simulink model "Final_V620140905h5b_fuben1"  (Simulink 7.9)
settings: Solver=FixedStepDiscrete  StartTime=0.0  StopTime=1  FixedStep=Auto  RelTol=1e-3
undefined symbols (not defined in the file or in its folder): Down, Up
libraries: tiiqmathlib x157, idelinklib_common x83, c2833xlib x37, simulink x12, c28xdmclib x12, c280xlib x7, simulink_extras x4, commutil2 x2, idelinklib_tgtpref x1, idelinklib_ticcs x1
(part 2 of 7)

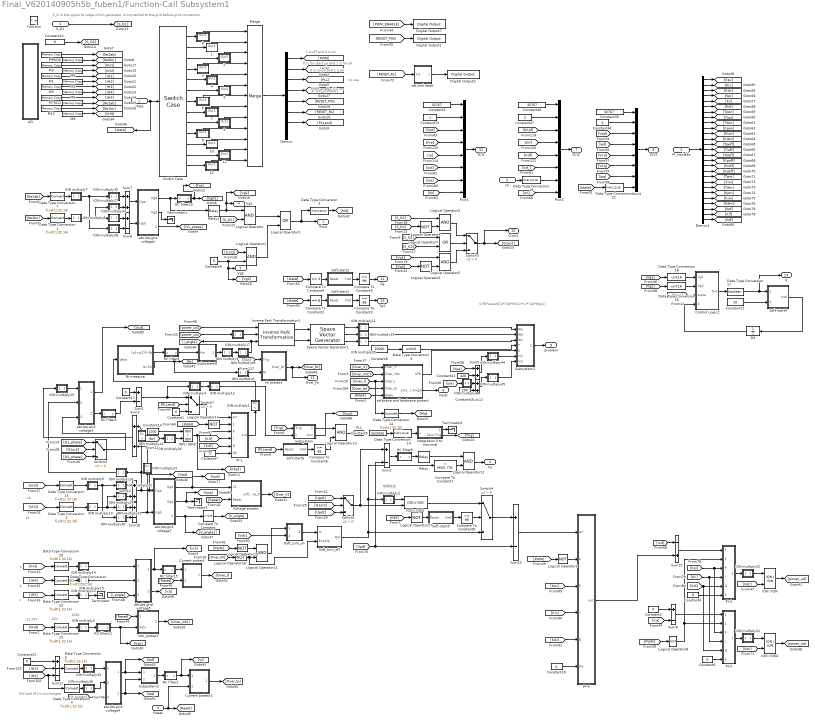
== system Final_V620140905h5b_fuben1/Function-Call Subsystem1 ==
  note: 1 is off and 0 is on
  note: 0 is for start up and 1 is for pll
  note: 0 is no pll and 1 is pll
  note: 21.25V
  note: 42V
  note: 1656
  note: PWM enable 1 is on
  note: S_G is the signal to judge which generator is connected to the grid before grid connection
  note: a
  note: b
  note: c
  note: no use
  note: IH2 and IH1 is exchanged.
  note: 0.95*squart[(2*740*Md)2+(2*740*Mq)2]
  note: cb
  note: ac
  note: 电网软启
  state : Inport
  PI_variable : Inport  Port=2
  Reset : Inport  Port=3
  S_G1 : Inport  Port=4
  ch : Inport  Port=5
  function : TriggerPort  TriggerType=function-call
  0 : Subsystem  TreatAsAtomicUnit=on
  1 : Subsystem  TreatAsAtomicUnit=on
  10 : Subsystem  TreatAsAtomicUnit=on
  11 : Subsystem  TreatAsAtomicUnit=on
  12 : Subsystem  TreatAsAtomicUnit=on
  2 : Subsystem  TreatAsAtomicUnit=on
  3 : Subsystem  TreatAsAtomicUnit=on
  4 : Subsystem  TreatAsAtomicUnit=on
  5 : Subsystem  TreatAsAtomicUnit=on
  6 : Subsystem  TreatAsAtomicUnit=on
  7 : Subsystem  TreatAsAtomicUnit=on
  8 : Subsystem  TreatAsAtomicUnit=on
  9 : Subsystem  TreatAsAtomicUnit=on
  AD : Subsystem  Priority=1
  Compare To Constant : simulink/Logic and Bit Operations/Compare To Constant  relop=>  const=0.8  OutDataTypeStr=uint8
  Compare To Constant1 : simulink/Logic and Bit Operations/Compare To Constant  relop=>  const=560/1.732  OutDataTypeStr=uint8
  Compare To Constant2 : simulink/Logic and Bit Operations/Compare To Constant  relop===  const=8  OutDataTypeStr=boolean
  Compare To Constant3 : simulink/Logic and Bit Operations/Compare To Constant  relop=>=  const=99  OutDataTypeStr=boolean
  Compare To Constant4 : simulink/Logic and Bit Operations/Compare To Constant  relop===  const=3  OutDataTypeStr=boolean
  Compare To Constant5 : simulink/Logic and Bit Operations/Compare To Constant  relop=>=  const=99  OutDataTypeStr=boolean
  Compare To Constant6 : simulink/Logic and Bit Operations/Compare To Constant  relop=>=  const=99  OutDataTypeStr=boolean
  Compare To Constant9 : simulink/Logic and Bit Operations/Compare To Constant  relop=<=  const=99  OutDataTypeStr=boolean
  Constant{1..2,4,6..7,17..18} (7 alike) : Constant  Value=0  OutDataTypeStr=fixdt(1,32,16)
  Constant11 : Constant  Value=10  OutDataTypeStr=fixdt(1,32,16)
  Constant12 : Constant  Value=0  OutDataTypeStr=boolean
  Constant13 : Constant  OutDataTypeStr=fixdt(1,32,16)
  Constant14 : Constant  Value=1200  OutDataTypeStr=fixdt(1,32,16)
  Constant16 : Constant  Value=100  OutDataTypeStr=fixdt(1,32,16)
  Constant21 : Constant  Value=420  OutDataTypeStr=fixdt(1,32,16)
  Constant23 : Constant  Value=0  OutDataTypeStr=fixdt(1,32,16)  SampleTime=-1
  Constant3 : Constant  Value=32767  OutDataTypeStr=fixdt(1,32,16)
  Constant30 : Constant  Value=32767  OutDataTypeStr=fixdt(1,32,16)
  Constant44 : Constant  Value=3  OutDataTypeStr=fixdt(1,32,16)
  Constant46 : Constant  Value=32767  OutDataTypeStr=fixdt(1,32,16)
  Constant47 : Constant  Value=2  OutDataTypeStr=fixdt(1,32,16)
  Constant5 : Constant  Value=50/5000  OutDataTypeStr=double
  Constant8 : Constant  Value=15000  OutDataTypeStr=int16
  Constant9 : Constant  Value=0  OutDataTypeStr=Inherit: Inherit via back propagation
  Control Logic2 : Stateflow chart  TreatAsAtomicUnit=on
  Current protect : Subsystem
  Current protect1 : Subsystem
  D5 : UnitDelay  SampleTime=-1
  Data Type Conversion{1..2,4..7,12..15,19..23} (15 alike) : DataTypeConversion  OutDataTypeStr=fixdt(1,32,16)
  Data Type Conversion16 : DataTypeConversion  OutDataTypeStr=uint16
  Data Type Conversion17 : DataTypeConversion  OutDataTypeStr=boolean
  Data Type Conversion18 : DataTypeConversion  OutDataTypeStr=uint16
  Data Type Conversion3 : DataTypeConversion  OutDataTypeStr=uint16
  Demux : Demux  Outputs=8
  Demux1 : Demux  Outputs=27
  Digital Output1 : c2833xlib/Digital Output  Priority=1  GPIO_Number=GPIO48~GPIO55  GPIO_Bit0=off  GPIO_BIT0_Toggle=off  GPIO_Bit1=on  GPIO_BIT1_Toggle=off  GPIO_Bit2=off  GPIO_BIT2_Toggle=off  GPIO_Bit3=off  GPIO_BIT3_Toggle=off  GPIO_Bit4=off  GPIO_BIT4_Toggle=off  GPIO_Bit5=off  GPIO_BIT5_Toggle=off  GPIO_Bit6=off  GPIO_BIT6_Toggle=off  GPIO_Bit7=off  GPIO_BIT7_Toggle=off
  Digital Output2 : c2833xlib/Digital Output  Priority=1  GPIO_Number=GPIO48~GPIO55  GPIO_Bit0=on  GPIO_BIT0_Toggle=off  GPIO_Bit1=off  GPIO_BIT1_Toggle=off  GPIO_Bit2=off  GPIO_BIT2_Toggle=off  GPIO_Bit3=off  GPIO_BIT3_Toggle=off  GPIO_Bit4=off  GPIO_BIT4_Toggle=off  GPIO_Bit5=off  GPIO_BIT5_Toggle=off  GPIO_Bit6=off  GPIO_BIT6_Toggle=off  GPIO_Bit7=off  GPIO_BIT7_Toggle=off
  Digital Output7 : c2833xlib/Digital Output  Priority=1  GPIO_Number=GPIO16~GPIO23  GPIO_Bit0=off  GPIO_BIT0_Toggle=off  GPIO_Bit1=off  GPIO_BIT1_Toggle=off  GPIO_Bit2=off  GPIO_BIT2_Toggle=off  GPIO_Bit3=on  GPIO_BIT3_Toggle=off  GPIO_Bit4=off  GPIO_BIT4_Toggle=off  GPIO_Bit5=off  GPIO_BIT5_Toggle=off  GPIO_Bit6=off  GPIO_BIT6_Toggle=off  GPIO_Bit7=off  GPIO_BIT7_Toggle=off
  ION multiply1 : Subsystem  mask{x=1/50}
      mask prompts: x "gain"
  ION multiply10 : Subsystem  mask{x=0.02536*50/29.6/1.0181}
      mask prompts: x "gain"
  ION multiply11 : Subsystem  mask{x=-1}
      mask prompts: x "gain"
  ION multiply12 : Subsystem  mask{x=1/100}
      mask prompts: x "gain"
  ION multiply13 : Subsystem  mask{x=0.0086*75/38}
      mask prompts: x "gain"
  ION multiply14 : Subsystem  mask{x=0.0086*75/38}
      mask prompts: x "gain"
  ION multiply15 : Subsystem  mask{x=0.0086*75/38}
      mask prompts: x "gain"
  ION multiply16 : Subsystem  mask{x=-1}
      mask prompts: x "gain"
  ION multiply17 : Subsystem  mask{x=-1}
      mask prompts: x "gain"
  ION multiply19 : Subsystem  mask{x=-1}
      mask prompts: x "gain"
  ION multiply2 : Subsystem  mask{x=1/327}
      mask prompts: x "gain"
  ION multiply20 : Subsystem  mask{x=-1}
      mask prompts: x "gain"
  ION multiply21 : Subsystem  mask{x=750/1000}
      mask prompts: x "gain"
  ION multiply22 : Subsystem  mask{x=750/1000}
      mask prompts: x "gain"
  ION multiply23 : Subsystem  mask{x=-1}
      mask prompts: x "gain"
  ION multiply24 : Subsystem  mask{x=-1}
      mask prompts: x "gain"
  ION multiply25 : Subsystem  mask{x=-1}
      mask prompts: x "gain"
  ION multiply26 : Subsystem  mask{x=10}
      mask prompts: x "gain"
  ION multiply27 : Subsystem  mask{x=1/3}
      mask prompts: x "gain"
  ION multiply28 : Subsystem  mask{x=1/3}
      mask prompts: x "gain"
  ION multiply29 : Subsystem  mask{x=1/3}
      mask prompts: x "gain"
  ION multiply3 : Subsystem  mask{x=0.04016*305/298}
      mask prompts: x "gain"
  ION multiply30 : Subsystem  mask{x=1/3}
      mask prompts: x "gain"
  ION multiply31 : Subsystem  mask{x=1/3}
      mask prompts: x "gain"
  ION multiply32 : Subsystem  mask{x=2/3}
      mask prompts: x "gain"
  ION multiply33 : Subsystem  mask{x=-0.0086*75/38}
      mask prompts: x "gain"
  ION multiply34 : Subsystem  mask{x=1/3}
      mask prompts: x "gain"
  ION multiply35 : Subsystem  mask{x=2/3}
      mask prompts: x "gain"
  ION multiply36 : Subsystem  mask{x=-0.0086*75/38}
      mask prompts: x "gain"
  ION multiply39 : Subsystem  mask{x=1/100}
      mask prompts: x "gain"
  ION multiply4 : Subsystem  mask{x=1/50}
      mask prompts: x "gain"
  ION multiply44 : Subsystem  mask{x=1/8}
      mask prompts: x "gain"
  ION multiply45 : Subsystem  mask{x=0}
      mask prompts: x "gain"
  ION multiply46 : Subsystem  mask{x=-1}
      mask prompts: x "gain"
  ION multiply5 : Subsystem  mask{x=1/50}
      mask prompts: x "gain"
  ION multiply6 : Subsystem  mask{x=10}
      mask prompts: x "gain"
  ION multiply7 : Subsystem  mask{x=-0.02436}
      mask prompts: x "gain"
  ION multiply8 : Subsystem  mask{x=-0.02436}
      mask prompts: x "gain"
  ION multiply9 : Subsystem  mask{x=0.02536*50/29.6/1.0181}
      mask prompts: x "gain"
  IQN / IQN : tiiqmathlib/IQN // IQN
  IQN / IQN2 : tiiqmathlib/IQN // IQN
  IQN / IQN3 : tiiqmathlib/IQN // IQN
  IQN x IQN1 : tiiqmathlib/IQN x IQN  multiplyOption=Multiply
  Integration 0 to maximal : Subsystem  mask{a=1}
      mask prompts: a "the maximal y"
  Inverse Park Transformation1 : c28xdmclib/Inverse Park Transformation
  Logical Operator{,1,3,5,11..13} (7 alike) : Logic  AllPortsSameDT=off  OutDataTypeStr=boolean
  Logical Operator{8..10,14,16} (5 alike) : Logic  Operator=NOT  Inputs=1  AllPortsSameDT=off  OutDataTypeStr=boolean
  Logical Operator17 : Logic  Operator=NOT  AllPortsSameDT=off  OutDataTypeStr=boolean
  Logical Operator2 : Logic  Operator=OR  AllPortsSameDT=off  OutDataTypeStr=boolean
  Logical Operator4 : Logic  Operator=NOT  AllPortsSameDT=off  OutDataTypeStr=boolean
  Logical Operator6 : Logic  Operator=NOT  AllPortsSameDT=off  OutDataTypeStr=boolean
  Logical Operator7 : Logic  Operator=OR  AllPortsSameDT=off  OutDataTypeStr=boolean
  M1 : idelinklib_common/Memory Copy  Priority=2  copyFrom=Specified source code symbol  copyFromAddressSource=Specify via dialog  copyFromAddress=M1  copyFromSrcCode=M1  dataTypeFrom=int16  dataDimensionFrom=1  useOffsetFrom=off  offsetFromSrc=Specify via dialog  offsetFrom=0  strideFrom=1  copyTo=Output port  copyToAddressSource=Specify via dialog  copyToAddress=temp  copyToSrcCode=M7  dataTypeTo=int16  useOffsetTo=on  offsetToSrc=Specify via dialog  offsetTo=0  strideTo=1  sampleTime=inf  useInitValue=off  initValueSrc=Specify constant value  initValue=bin2dec('00000000')  initValueSrcCode=myInitValueVariable  useAsMask=off  maskOperator=bitwise AND  useTermValue=off  termValue=bin2dec('00000000')  isRealtimeEnabled=off  emitCCBeforeWrite=off  CCBeforeWrite=/* Custom Code Before Write*/  emitCCAfterWrite=off  CCAfterWrite=/* Custom Code After Write*/  useDMACopy=off  enableBlockingMode=off
  M10 : idelinklib_common/Memory Copy  Priority=2  copyFrom=Specified source code symbol  copyFromAddressSource=Specify via dialog  copyFromAddress=M1  copyFromSrcCode=M10  dataTypeFrom=int16  dataDimensionFrom=1  useOffsetFrom=off  offsetFromSrc=Specify via dialog  offsetFrom=0  strideFrom=1  copyTo=Output port  copyToAddressSource=Specify via dialog  copyToAddress=temp  copyToSrcCode=M7  dataTypeTo=int16  useOffsetTo=on  offsetToSrc=Specify via dialog  offsetTo=0  strideTo=1  sampleTime=inf  useInitValue=off  initValueSrc=Specify constant value  initValue=bin2dec('00000000')  initValueSrcCode=myInitValueVariable  useAsMask=off  maskOperator=bitwise AND  useTermValue=off  termValue=bin2dec('00000000')  isRealtimeEnabled=off  emitCCBeforeWrite=off  CCBeforeWrite=/* Custom Code Before Write*/  emitCCAfterWrite=off  CCAfterWrite=/* Custom Code After Write*/  useDMACopy=off  enableBlockingMode=off
  M11 : idelinklib_common/Memory Copy  Priority=2  copyFrom=Specified source code symbol  copyFromAddressSource=Specify via dialog  copyFromAddress=M1  copyFromSrcCode=M11  dataTypeFrom=int16  dataDimensionFrom=1  useOffsetFrom=off  offsetFromSrc=Specify via dialog  offsetFrom=0  strideFrom=1  copyTo=Output port  copyToAddressSource=Specify via dialog  copyToAddress=temp  copyToSrcCode=M7  dataTypeTo=int16  useOffsetTo=on  offsetToSrc=Specify via dialog  offsetTo=0  strideTo=1  sampleTime=inf  useInitValue=off  initValueSrc=Specify constant value  initValue=bin2dec('00000000')  initValueSrcCode=myInitValueVariable  useAsMask=off  maskOperator=bitwise AND  useTermValue=off  termValue=bin2dec('00000000')  isRealtimeEnabled=off  emitCCBeforeWrite=off  CCBeforeWrite=/* Custom Code Before Write*/  emitCCAfterWrite=off  CCAfterWrite=/* Custom Code After Write*/  useDMACopy=off  enableBlockingMode=off
  M12 : idelinklib_common/Memory Copy  Priority=2  copyFrom=Specified source code symbol  copyFromAddressSource=Specify via dialog  copyFromAddress=M1  copyFromSrcCode=M12  dataTypeFrom=int16  dataDimensionFrom=1  useOffsetFrom=off  offsetFromSrc=Specify via dialog  offsetFrom=0  strideFrom=1  copyTo=Output port  copyToAddressSource=Specify via dialog  copyToAddress=temp  copyToSrcCode=M7  dataTypeTo=int16  useOffsetTo=on  offsetToSrc=Specify via dialog  offsetTo=0  strideTo=1  sampleTime=inf  useInitValue=off  initValueSrc=Specify constant value  initValue=bin2dec('00000000')  initValueSrcCode=myInitValueVariable  useAsMask=off  maskOperator=bitwise AND  useTermValue=off  termValue=bin2dec('00000000')  isRealtimeEnabled=off  emitCCBeforeWrite=off  CCBeforeWrite=/* Custom Code Before Write*/  emitCCAfterWrite=off  CCAfterWrite=/* Custom Code After Write*/  useDMACopy=off  enableBlockingMode=off
  M2 : idelinklib_common/Memory Copy  Priority=2  copyFrom=Specified source code symbol  copyFromAddressSource=Specify via dialog  copyFromAddress=M1  copyFromSrcCode=M2  dataTypeFrom=int16  dataDimensionFrom=1  useOffsetFrom=off  offsetFromSrc=Specify via dialog  offsetFrom=0  strideFrom=1  copyTo=Output port  copyToAddressSource=Specify via dialog  copyToAddress=temp  copyToSrcCode=M7  dataTypeTo=int16  useOffsetTo=on  offsetToSrc=Specify via dialog  offsetTo=0  strideTo=1  sampleTime=inf  useInitValue=off  initValueSrc=Specify constant value  initValue=bin2dec('00000000')  initValueSrcCode=myInitValueVariable  useAsMask=off  maskOperator=bitwise AND  useTermValue=off  termValue=bin2dec('00000000')  isRealtimeEnabled=off  emitCCBeforeWrite=off  CCBeforeWrite=/* Custom Code Before Write*/  emitCCAfterWrite=off  CCAfterWrite=/* Custom Code After Write*/  useDMACopy=off  enableBlockingMode=off
  M3 : idelinklib_common/Memory Copy  Priority=2  copyFrom=Specified source code symbol  copyFromAddressSource=Specify via dialog  copyFromAddress=M1  copyFromSrcCode=M3  dataTypeFrom=int16  dataDimensionFrom=1  useOffsetFrom=off  offsetFromSrc=Specify via dialog  offsetFrom=0  strideFrom=1  copyTo=Output port  copyToAddressSource=Specify via dialog  copyToAddress=temp  copyToSrcCode=M7  dataTypeTo=int16  useOffsetTo=on  offsetToSrc=Specify via dialog  offsetTo=0  strideTo=1  sampleTime=inf  useInitValue=off  initValueSrc=Specify constant value  initValue=bin2dec('00000000')  initValueSrcCode=myInitValueVariable  useAsMask=off  maskOperator=bitwise AND  useTermValue=off  termValue=bin2dec('00000000')  isRealtimeEnabled=off  emitCCBeforeWrite=off  CCBeforeWrite=/* Custom Code Before Write*/  emitCCAfterWrite=off  CCAfterWrite=/* Custom Code After Write*/  useDMACopy=off  enableBlockingMode=off
  M4 : idelinklib_common/Memory Copy  Priority=2  copyFrom=Specified source code symbol  copyFromAddressSource=Specify via dialog  copyFromAddress=M1  copyFromSrcCode=M4  dataTypeFrom=int16  dataDimensionFrom=1  useOffsetFrom=off  offsetFromSrc=Specify via dialog  offsetFrom=0  strideFrom=1  copyTo=Output port  copyToAddressSource=Specify via dialog  copyToAddress=temp  copyToSrcCode=M7  dataTypeTo=int16  useOffsetTo=on  offsetToSrc=Specify via dialog  offsetTo=0  strideTo=1  sampleTime=inf  useInitValue=off  initValueSrc=Specify constant value  initValue=bin2dec('00000000')  initValueSrcCode=myInitValueVariable  useAsMask=off  maskOperator=bitwise AND  useTermValue=off  termValue=bin2dec('00000000')  isRealtimeEnabled=off  emitCCBeforeWrite=off  CCBeforeWrite=/* Custom Code Before Write*/  emitCCAfterWrite=off  CCAfterWrite=/* Custom Code After Write*/  useDMACopy=off  enableBlockingMode=off
  M5 : idelinklib_common/Memory Copy  Priority=2  copyFrom=Specified source code symbol  copyFromAddressSource=Specify via dialog  copyFromAddress=M1  copyFromSrcCode=M5  dataTypeFrom=int16  dataDimensionFrom=1  useOffsetFrom=off  offsetFromSrc=Specify via dialog  offsetFrom=0  strideFrom=1  copyTo=Output port  copyToAddressSource=Specify via dialog  copyToAddress=temp  copyToSrcCode=M7  dataTypeTo=int16  useOffsetTo=on  offsetToSrc=Specify via dialog  offsetTo=0  strideTo=1  sampleTime=inf  useInitValue=off  initValueSrc=Specify constant value  initValue=bin2dec('00000000')  initValueSrcCode=myInitValueVariable  useAsMask=off  maskOperator=bitwise AND  useTermValue=off  termValue=bin2dec('00000000')  isRealtimeEnabled=off  emitCCBeforeWrite=off  CCBeforeWrite=/* Custom Code Before Write*/  emitCCAfterWrite=off  CCAfterWrite=/* Custom Code After Write*/  useDMACopy=off  enableBlockingMode=off
  M6 : idelinklib_common/Memory Copy  Priority=2  copyFrom=Specified source code symbol  copyFromAddressSource=Specify via dialog  copyFromAddress=M1  copyFromSrcCode=M6  dataTypeFrom=int16  dataDimensionFrom=1  useOffsetFrom=off  offsetFromSrc=Specify via dialog  offsetFrom=0  strideFrom=1  copyTo=Output port  copyToAddressSource=Specify via dialog  copyToAddress=temp  copyToSrcCode=M7  dataTypeTo=int16  useOffsetTo=on  offsetToSrc=Specify via dialog  offsetTo=0  strideTo=1  sampleTime=inf  useInitValue=off  initValueSrc=Specify constant value  initValue=bin2dec('00000000')  initValueSrcCode=myInitValueVariable  useAsMask=off  maskOperator=bitwise AND  useTermValue=off  termValue=bin2dec('00000000')  isRealtimeEnabled=off  emitCCBeforeWrite=off  CCBeforeWrite=/* Custom Code Before Write*/  emitCCAfterWrite=off  CCAfterWrite=/* Custom Code After Write*/  useDMACopy=off  enableBlockingMode=off
  M7 : idelinklib_common/Memory Copy  Priority=2  copyFrom=Specified source code symbol  copyFromAddressSource=Specify via dialog  copyFromAddress=M1  copyFromSrcCode=M7  dataTypeFrom=int16  dataDimensionFrom=1  useOffsetFrom=off  offsetFromSrc=Specify via dialog  offsetFrom=0  strideFrom=1  copyTo=Output port  copyToAddressSource=Specify via dialog  copyToAddress=temp  copyToSrcCode=M7  dataTypeTo=int16  useOffsetTo=on  offsetToSrc=Specify via dialog  offsetTo=0  strideTo=1  sampleTime=inf  useInitValue=off  initValueSrc=Specify constant value  initValue=bin2dec('00000000')  initValueSrcCode=myInitValueVariable  useAsMask=off  maskOperator=bitwise AND  useTermValue=off  termValue=bin2dec('00000000')  isRealtimeEnabled=off  emitCCBeforeWrite=off  CCBeforeWrite=/* Custom Code Before Write*/  emitCCAfterWrite=off  CCAfterWrite=/* Custom Code After Write*/  useDMACopy=off  enableBlockingMode=off
  M8 : idelinklib_common/Memory Copy  Priority=2  copyFrom=Specified source code symbol  copyFromAddressSource=Specify via dialog  copyFromAddress=M1  copyFromSrcCode=M8  dataTypeFrom=int16  dataDimensionFrom=1  useOffsetFrom=off  offsetFromSrc=Specify via dialog  offsetFrom=0  strideFrom=1  copyTo=Output port  copyToAddressSource=Specify via dialog  copyToAddress=temp  copyToSrcCode=M7  dataTypeTo=int16  useOffsetTo=on  offsetToSrc=Specify via dialog  offsetTo=0  strideTo=1  sampleTime=inf  useInitValue=off  initValueSrc=Specify constant value  initValue=bin2dec('00000000')  initValueSrcCode=myInitValueVariable  useAsMask=off  maskOperator=bitwise AND  useTermValue=off  termValue=bin2dec('00000000')  isRealtimeEnabled=off  emitCCBeforeWrite=off  CCBeforeWrite=/* Custom Code Before Write*/  emitCCAfterWrite=off  CCAfterWrite=/* Custom Code After Write*/  useDMACopy=off  enableBlockingMode=off
  M9 : idelinklib_common/Memory Copy  Priority=2  copyFrom=Specified source code symbol  copyFromAddressSource=Specify via dialog  copyFromAddress=M1  copyFromSrcCode=M9  dataTypeFrom=int16  dataDimensionFrom=1  useOffsetFrom=off  offsetFromSrc=Specify via dialog  offsetFrom=0  strideFrom=1  copyTo=Output port  copyToAddressSource=Specify via dialog  copyToAddress=temp  copyToSrcCode=M7  dataTypeTo=int16  useOffsetTo=on  offsetToSrc=Specify via dialog  offsetTo=0  strideTo=1  sampleTime=inf  useInitValue=off  initValueSrc=Specify constant value  initValue=bin2dec('00000000')  initValueSrcCode=myInitValueVariable  useAsMask=off  maskOperator=bitwise AND  useTermValue=off  termValue=bin2dec('00000000')  isRealtimeEnabled=off  emitCCBeforeWrite=off  CCBeforeWrite=/* Custom Code Before Write*/  emitCCAfterWrite=off  CCAfterWrite=/* Custom Code After Write*/  useDMACopy=off  enableBlockingMode=off
  Merge : Merge  Inputs=13
  Mux1 : Mux  Inputs=8
  Mux2 : Mux  Inputs=8
  Mux3 : Mux  Inputs=8
  Nr measure : Subsystem
  Nr protect : Subsystem
  PI-1 : Subsystem  mask{ermax=200, ermin=-200, max=150, min=-150}
      mask prompts: ermax "Err max limit"; ermin "Err min limit"; max "Output max limit"; min "Output min limit"
  PI-3 : Subsystem  mask{ermax=500, ermin=-500, max=500, min=-500}
      mask prompts: ermax "Err max limit"; ermin "Err min limit"; max "Output max limit"; min "Output min limit"
  PI-4 : Subsystem  mask{ermax=500, ermin=-500, max=165, min=0}
      mask prompts: ermax "Err max limit"; ermin "Err min limit"; max "Output max limit"; min "Output min limit"
  PI-5 : Subsystem  mask{ermax=500, ermin=-500, max=500, min=-500}
      mask prompts: ermax "Err max limit"; ermin "Err min limit"; max "Output max limit"; min "Output min limit"
  RC filter10 : Subsystem  mask{a=0.01}
      mask prompts: a "Time Constant"
  RC filter11 : Subsystem  mask{a=0.01}
      mask prompts: a "Time Constant"
  RC filter15 : Subsystem  mask{a=0.1}
      mask prompts: a "Time Constant"
  RC filter2 : Subsystem  mask{a=0.5}
      mask prompts: a "Time Constant"
  RC filter3 : Subsystem  mask{a=0.5}
      mask prompts: a "Time Constant"
  RC filter4 : Subsystem  mask{a=0.8}
      mask prompts: a "Time Constant"
  RC filter9 : Subsystem  mask{a=0.8}
      mask prompts: a "Time Constant"
  Relay : Relay  OnSwitchValue=20  OffSwitchValue=10  OnOutputValue=0  OffOutputValue=1
  Relay1 : Relay  OnSwitchValue=300  OffSwitchValue=250
  Soft-start1 : Subsystem  mask{a=0.02/0.2, b=100}
      mask prompts: a "soft time"; b "Vref"
  Soft-start2 : Subsystem  mask{a=0.02/0.01, b=100}
      mask prompts: a "soft time"; b "Vref"
  Soft-start4 : Subsystem
  Soft-start5 : Subsystem  mask{a=0.02/2, b=100}
      mask prompts: a "soft time"; b "Vref"
  Soft-start6 : Subsystem  mask{a=0.02/6, b=100}
      mask prompts: a "soft time"; b "Vref"
  Soft_turn_off : Subsystem
  Soft_turn_on : Subsystem
  Space Vector Generator1 : c28xdmclib/Space Vector Generator
  Subsystem : Subsystem
  Subsystem1 : Subsystem
  Subsystem2 : Subsystem
  Subsystem8 : Subsystem
  Sum{1..2,6,9..10,13} (6 alike) : Sum  Inputs=+-
  Sum{3,5,7,12,17} (5 alike) : Sum
  Sum15 : Sum  Inputs=-+
  Sum21 : Sum  Inputs=+--
  Switch Case : SwitchCase  CaseConditions={0,1,2,3,4,5,6,7,8,9,10,11,12}  ShowDefaultCase=off
  Switch{1..4,7} (5 alike) : Switch  Criteria=u2 > Threshold  SaturateOnIntegerOverflow=on  InputSameDT=on
  Terminator{,1..3} (4 alike) : Terminator
  Vdc_protect : Subsystem
  Voltage protect : Subsystem
  abc/dq-grid voltage1 : Subsystem
  abc/dq-grid voltage3 : Subsystem
  abc/dq-grid voltage4 : Subsystem
  abc/dq-grid voltage5 : Subsystem
  abc/dq-grid voltage7 : Subsystem
  set and reset : Subsystem
  softwave and hardwave protect : Subsystem
  Vbus : Outport
  Vs : Outport  Port=2
  PLL : Outport  Port=3
  Vg1 : Outport  Port=4
  Vg2 : Outport  Port=5
  Fault : Outport  Port=6
  SCI2 : Outport  Port=7
  SCI3 : Outport  Port=8
  problem : Outport  Port=9
  G1or2 : Outport  Port=10
  Sg : Outport  Port=11
  SCI1 : Outport  Port=12
  Over_Nr : Outport  Port=13
  K : Outport  Port=14
  Sg1 : Outport  Port=15
  wires:
  Inverse Park Transformation1/1 -> Space Vector Generator1/1
  Inverse Park Transformation1/2 -> Space Vector Generator1/2
  Subsystem8/1(angle) -> ION multiply5/1(x)
  [No1ab] -> Data Type Conversion7/1
  [No1bc] -> Data Type Conversion1/1
  abc/dq-grid voltage1/1(Ugd) -> RC filter10/1(x), Relay1/1
  Switch Case/1 -> 0/Action
  1/1(Out1) -> Merge/2
  2/1(Out1) -> Merge/3
  3/1(Out1) -> Merge/4
  4/1(Out1) -> Merge/5
  5/1(Out1) -> Merge/6
  Merge/1 -> Demux/1
  Demux/1 -> [PWM]
  Demux/2 -> [REF]
  state/1 -> Switch Case/1, [state]
  Demux/3 -> [PLL]
  Relay1/1 -> Logical Operator/1, Vg1/1, [Vg1]
  [S_G1] -> Logical Operator/2
  Logical Operator/1 -> Logical Operator2/1
  Logical Operator2/1 -> Vbus/1, Data Type Conversion5/1
  Constant12/1 -> [S_G2]
  [S_G1] -> Logical Operator3/1
  Logical Operator4/1 -> Logical Operator3/2
  [S_G2] -> Logical Operator4/1
  [G1or2] -> Switch1/2
  [Ugd2] -> Switch1/3
  [Ugd1] -> Switch1/1
  [Vg1] -> Logical Operator5/1
  Logical Operator6/1 -> Logical Operator5/2
  [Vg2] -> Logical Operator6/1
  Switch3/1 -> [G1or2], G1or2/1
  Logical Operator7/1 -> Switch3/2
  [S_G1] -> Logical Operator7/1
  [S_G2] -> Logical Operator7/2
  6/1(Out1) -> Merge/7
  Logical Operator3/1 -> Switch3/1
  Logical Operator5/1 -> Switch3/3
  Data Type Conversion1/1 -> ION multiply8/1(x)
  Data Type Conversion7/1 -> ION multiply7/1(x)
  [PWM_ENABLE] -> Digital Output7/1
  Demux/4 -> [PWM_ENABLE]
  [RESET_PIN] -> Digital Output1/1
  Demux/5 -> [RESET_PIN]
  Demux/6 -> [RESET_RL]
  Space Vector Generator1/1 -> ION multiply11/1(x)
  Space Vector Generator1/2 -> ION multiply19/1(x)
  Space Vector Generator1/3 -> ION multiply20/1(x)
  Data Type Conversion2/1 -> ION multiply10/1(x)
  Data Type Conversion13/1 -> ION multiply9/1(x)
  ION multiply10/1(Kx) -> ION multiply29/1(x), ION multiply31/1(x)
  [VH2] -> Data Type Conversion13/1
  [VH1] -> Data Type Conversion2/1
  [IH3] -> Data Type Conversion20/1
  [IH4] -> Data Type Conversion21/1
  Data Type Conversion21/1 -> ION multiply13/1(x)
  Data Type Conversion20/1 -> ION multiply14/1(x)
  [IH5] -> Data Type Conversion23/1
  Data Type Conversion23/1 -> ION multiply15/1(x)
  abc/dq-grid voltage5/1(igd) -> RC filter15/1(x), [icd]
  [i_angle] -> abc/dq-grid voltage5/3(angle)
  RC filter15/1(y) -> Current protect/1(igdin)
  7/1(Out1) -> Merge/8
  Mux2/1 -> SCI2/1
  Constant30/1 -> Mux3/1
  Constant44/1 -> Mux3/2
  Mux3/1 -> SCI3/1
  Constant46/1 -> Mux2/1
  Constant47/1 -> Mux2/2
  Subsystem1/1(Out1) -> problem/1
  [on] -> Mux2/8
  Switch4/1 -> Sum13/1
  Voltage protect/1(softwave_V) -> [Over_V]
  [Reset] -> Voltage protect/2(Reset)
  [Reset] -> Current protect/2(Reset)
  Current protect/1(Software_I) -> [Over_I]
  Sum2/1 -> RC filter9/1(x)
  RC filter9/1(y) -> Relay/1
  Constant5/1 -> Data Type Conversion14/1
  Data Type Conversion14/1 -> Integration 0 to maximal/1(x)
  Integration 0 to maximal/2(Zero Trig) -> [Trig]
  [Over_V] -> softwave and hardwave protect/1(Over_V)
  RC filter10/1(y) -> [Ugd1], [Fre]
  [VH9] -> Data Type Conversion15/1
  Data Type Conversion15/1 -> ION multiply3/1(x)
  ION multiply3/1(Kx) -> RC filter11/1(x)
  RC filter11/1(y) -> Vdc_protect/2(Vdin), [Vdc]
  [Over_Vdc] -> softwave and hardwave protect/2(Over_Vdc)
  Compare To Constant/1 -> [V_angle]
  [Reset] -> Vdc_protect/1(Reset)
  Vdc_protect/1(Vdguoya) -> [Over_Vdc]
  Switch Case/9 -> 8/Action
  8/1(Out1) -> Merge/9
  Switch Case/8 -> 7/Action
  Switch Case/7 -> 6/Action
  Switch Case/6 -> 5/Action
  Switch Case/5 -> 4/Action
  Switch Case/4 -> 3/Action
  Switch Case/3 -> 2/Action
  Switch Case/2 -> 1/Action
  Demux/7 -> [PLLend]
  Switch Case/10 -> 9/Action
  9/1(Out1) -> Merge/10
  0/1(Out1) -> Merge/1
  10/1(Out1) -> Merge/11
  11/1(Out1) -> Merge/12
  Switch Case/12 -> 11/Action
  Switch Case/13 -> 12/Action
  12/1(Out1) -> Merge/13
  [Over_I] -> softwave and hardwave protect/3(Over_I), Data Type Conversion12/1
  abc/dq-grid voltage5/2(igq) -> [icq]
  ION multiply14/1(Kx) -> abc/dq-grid voltage5/1(iga)
  ION multiply13/1(Kx) -> abc/dq-grid voltage5/2(igb)
  ION multiply15/1(Kx) -> Terminator/1
  M1/1 -> [IH1]
  M2/1 -> [IH2]
  M3/1 -> [VH1]
  M4/1 -> [VH2]
  M5/1 -> [IH3]
  M6/1 -> [IH4]
  M7/1 -> [IH5]
  M8/1 -> [VH9]
  M11/1 -> [No1ab]
  M12/1 -> [No1bc]
  M9/1 -> [No2ab]
  M10/1 -> [No2bc]
  ION multiply11/1(Kx) -> Subsystem1/1(Wa)
  ION multiply19/1(Kx) -> Subsystem1/2(Wb)
  ION multiply20/1(Kx) -> Subsystem1/3(Wc)
  PI-3/1(out) -> ION multiply21/1(x)
  ION multiply21/1(Kx) -> IQN / IQN2/1
  ION multiply32/1(Kx) -> Sum12/1
  ION multiply29/1(Kx) -> Sum12/2
  ION multiply31/1(Kx) -> Sum10/1
  ION multiply30/1(Kx) -> Sum10/2
  Sum12/1 -> ION multiply16/1(x), ION multiply24/1(x), abc/dq-grid voltage7/1(Uga), [Vpa]
  Sum10/1 -> abc/dq-grid voltage7/2(Ugb), ION multiply23/1(x)
  abc/dq-grid voltage7/3(Phase) -> Compare To Constant/1, [V_angle1]
  abc/dq-grid voltage7/2(Ugq) -> Terminator3/1, [Vpq]
  Integration 0 to maximal/1(y) -> Terminator2/1
  [Vpd] -> Mux3/3
  [ipd] -> Mux3/4
  [Vcq] -> Mux3/6
  [ipq] -> Mux3/7
  abc/dq-grid voltage7/1(Ugd) -> Voltage protect/1(V1), [Vpd]
  [Vcd] -> Mux3/5
  [power_uq] -> ION multiply17/1(x)
  [power_ud] -> Inverse Park Transformation1/1
  [PWM] -> Logical Operator9/1
  Logical Operator10/1 -> Logical Operator11/1
  [PWM] -> Logical Operator10/1
  Switch1/1 -> IQN x IQN1/2, Sum2/1
  ION multiply2/1(Kx) -> IQN x IQN1/1
  IQN x IQN1/1 -> Switch4/1
  ION multiply22/1(Kx) -> IQN / IQN/1
  Logical Operator8/1 -> PI-5/2(reset), PI-3/2(reset)
  [PWM] -> Logical Operator8/1
  [Vdc] -> Soft_turn_on/2(Vdc)
  Switch Case/11 -> 10/Action
  set and reset/1(Out1) -> Digital Output2/1
  [RESET_RL] -> set and reset/1(In1)
  IQN / IQN/1 -> [power_ud]
  IQN / IQN2/1 -> [power_uq]
  [icd] -> Sum15/1
  [icq] -> Sum9/2
  PI-5/1(out) -> ION multiply22/1(x)
  Nr measure/2(Nr/10) -> [Nr], ION multiply6/1(x)
  [Kpi] -> PI-5/3(P), PI-3/3(P)
  [Kii] -> PI-5/4(I), PI-3/4(I)
  [Kdi] -> PI-5/5(D), PI-3/5(D)
  Sum15/1 -> PI-5/1(err)
  Sum9/1 -> PI-3/1(err)
  Compare To Constant1/1 -> Logical Operator12/2
  Logical Operator12/1 -> Vs/1
  Relay/1 -> Logical Operator12/1
  Logical Operator9/1 -> PI-4/2(reset)
  PI_variable/1 -> Demux1/1
  Demux1/1 -> [Kpv]
  Demux1/2 -> [Kiv]
  Demux1/3 -> [Kdv]
  Demux1/4 -> [Kpi]
  Demux1/5 -> [Kii]
  Demux1/6 -> [Kdi]
  Demux1/7 -> [Tpon]
  Demux1/8 -> [Tion]
  Demux1/9 -> [Tdon]
  Demux1/10 -> [Kpon]
  Demux1/11 -> [Kion]
  Demux1/12 -> [Kdon]
  Demux1/13 -> [Tpoff]
  Demux1/14 -> [Tioff]
  Demux1/15 -> [Tdoff]
  Demux1/16 -> [Kpoff]
  Demux1/17 -> [Kioff]
  Demux1/18 -> [Kdoff]
  Demux1/19 -> [Tpm]
  Demux1/20 -> [Tim]
  Demux1/21 -> [Tdm]
  Demux1/22 -> [Kpm]
  Demux1/23 -> [Kim]
  Demux1/24 -> [Kdm]
  Constant4/1 -> PI-5/6(OV)
  Constant6/1 -> PI-3/6(OV)
  Demux1/25 -> [Kpf]
  Demux1/26 -> [Kif]
  Demux1/27 -> [Kdf]
  Constant8/1 -> Data Type Conversion3/1
  [G1or2] -> Switch2/2
  [G1_phase] -> Switch2/1
  [G2_phase] -> Switch2/3
  Data Type Conversion3/1 -> Subsystem1/4(T)
  [Over_Ip] -> softwave and hardwave protect/4(Over_Ip)
  Constant2/1 -> Sum9/1
  Soft-start2/1(Vref) -> Compare To Constant5/1
  [state] -> Compare To Constant4/1
  Compare To Constant4/1 -> Soft-start2/1(Reset)
  Compare To Constant5/1 -> Sg/1
  [Vdc] -> IQN / IQN/2
  [Vdc] -> IQN / IQN2/2
  ION multiply9/1(Kx) -> ION multiply32/1(x), ION multiply30/1(x)
  [Vpd] -> Sum13/2, Sum2/2
  ION multiply8/1(Kx) -> ION multiply34/1(x), ION multiply27/1(x)
  ION multiply35/1(Kx) -> Sum7/1
  ION multiply27/1(Kx) -> Sum7/2
  ION multiply34/1(Kx) -> Sum6/1
  ION multiply28/1(Kx) -> Sum6/2
  Sum7/1 -> abc/dq-grid voltage1/1(Uga)
  Sum6/1 -> abc/dq-grid voltage1/2(Ugb)
  ION multiply7/1(Kx) -> ION multiply28/1(x), ION multiply35/1(x)
  abc/dq-grid voltage1/3(Phase) -> [G1_phase]
  abc/dq-grid voltage1/2(Ugq) -> Terminator1/1
  Sum13/1 -> PI-4/1(err)
  [PWM] -> Logical Operator14/1
  abc/dq-grid voltage4/1(igd) -> Subsystem2/1(In1), [ipd]
  abc/dq-grid voltage4/2(igq) -> Subsystem2/2(In2), [ipq]
  Current protect1/1(Software_I) -> [Over_Ip]
  RC filter2/1(y) -> Current protect1/1(igdin), [ip]
  PI-4/1(out) -> Sum15/2
  Subsystem2/1(Out1) -> RC filter2/1(x)
  Nr measure/1((p1+p2)Fr-Fp) -> RC filter4/1(x)
  [KKpf] -> Mux2/3
  [Kif] -> Mux2/4
  [Kdf] -> Mux2/5
  [icd_] -> Mux2/6
  Mux1/1 -> SCI1/1
  Constant3/1 -> Mux1/1
  Constant13/1 -> Mux1/2
  [Nr] -> Mux1/8
  [Vpd] -> Mux1/3
  [ip] -> Mux1/5
  [ipd] -> Mux1/6
  [ipq] -> Mux1/7
  [V_angle1] -> abc/dq-grid voltage4/3(angle)
  [Fre] -> Mux1/4
  ION multiply6/1(Kx) -> Nr protect/2(Nr)
  Reset/1 -> [Reset], Current protect1/2(Reset)
  Data Type Conversion5/1 -> [Md]
  [Trig] -> Nr protect/1(Trig)
  Nr protect/1(Over_Nr) -> [Over_Nr], Over_Nr/1
  Soft_turn_on/1(Out) -> Soft_turn_off/1(In)
  Soft_turn_off/1(Ref) -> Compare To Constant1/1, ION multiply2/1(x), Switch4/3
  [Over_Nr] -> Logical Operator16/1
  [PWM] -> softwave and hardwave protect/5(PWM)
  softwave and hardwave protect/2(protect singal) -> Fault/1
  Logical Operator11/1 -> Soft_turn_on/1(Enable)
  Logical Operator16/1 -> Logical Operator11/2, Soft_turn_off/2(Enable)
  S_G1/1 -> [S_G1]
  Constant11/1 -> Soft-start4/2(T)
  Control Logic2/1(Out) -> Data Type Conversion17/1
  Soft-start4/1(Vref) -> D5/1
  D5/1 -> Control Logic2/4(K)
  [state] -> Control Logic2/3(state)
  [Vg1] -> Data Type Conversion18/1
  [Vg2] -> Data Type Conversion16/1
  Data Type Conversion18/1 -> Control Logic2/1(Vg1)
  Data Type Conversion16/1 -> Control Logic2/2(Vg2)
  Data Type Conversion17/1 -> Soft-start4/1(Reset), K/1
  Data Type Conversion12/1 -> [Mq]
  ch/1 -> Data Type Conversion19/1
  Soft-start5/1(Vref) -> Compare To Constant9/1
  Logical Operator17/1 -> Soft-start5/1(Reset)
  [REF] -> Logical Operator17/1
  Compare To Constant9/1 -> Switch4/2
  Data Type Conversion19/1 -> Mux2/7
  Soft-start1/1(Vref) -> Compare To Constant3/1
  [state] -> Compare To Constant2/1
  Compare To Constant2/1 -> Soft-start1/1(Reset)
  Compare To Constant3/1 -> Sg1/1
  [state] -> Data Type Conversion22/1
  Data Type Conversion22/1 -> Mux3/8
  RC filter4/1(y) -> Subsystem8/1(fre)
  ION multiply5/1(Kx) -> ION multiply39/1(x)
  ION multiply39/1(Kx) -> Inverse Park Transformation1/3, [i_angle]
  Switch2/1 -> abc/dq-grid voltage3/3(angle)
  Logical Operator14/1 -> PI-1/2(reset)
  Constant17/1 -> Sum1/1
  Sum1/1 -> Switch7/1, ION multiply4/1(x)
  Constant1/1 -> Switch7/3
  abc/dq-grid voltage3/2(igq) -> RC filter3/1(x)
  [PLLend] -> Switch7/2
  Switch7/1 -> PI-1/1(err)
  PI-1/1(out) -> ION multiply1/1(x)
  abc/dq-grid voltage3/1(igd) -> [Vcd]
  Constant7/1 -> PI-1/6(OV)
  Constant9/1 -> Logical Operator1/2, Vg2/1, [Vg2]
  [S_G2] -> Logical Operator1/1
  Logical Operator1/1 -> Logical Operator2/2
  [Trig] -> Subsystem/1(Trig)
  Subsystem/1(On/off) -> Logical Operator13/1
  Logical Operator13/1 -> PLL/1
  Compare To Constant6/1 -> Logical Operator13/2
  Soft-start6/1(Vref) -> Compare To Constant6/1
  [PLLend] -> Soft-start6/1(Reset)
  RC filter3/1(y) -> Sum1/2
  ION multiply1/1(Kx) -> Nr measure/1(deta)
  Subsystem/2(sum) -> [Vcq]
  ION multiply4/1(Kx) -> ION multiply12/1(x)
  ION multiply12/1(Kx) -> Subsystem/2(x)
  ION multiply16/1(Kx) -> abc/dq-grid voltage3/2(igb)
  ION multiply23/1(Kx) -> Sum3/2
  ION multiply24/1(Kx) -> Sum3/1
  Sum3/1 -> ION multiply25/1(x)
  ION multiply25/1(Kx) -> abc/dq-grid voltage3/1(iga)
  [Kif] -> PI-1/4(I)
  [Kdf] -> PI-1/5(D)
  Constant14/1 -> IQN / IQN3/1
  [Nr] -> ION multiply26/1(x)
  ION multiply26/1(Kx) -> IQN / IQN3/2
  IQN / IQN3/1 -> PI-1/3(P), [KKpf]
  Data Type Conversion4/1 -> ION multiply36/1(x)
  Data Type Conversion6/1 -> ION multiply33/1(x)
  Constant23/1 -> Sum21/1
  [IH1] -> Sum21/2
  [IH2] -> Sum21/3, Data Type Conversion4/1
  Sum21/1 -> Data Type Conversion6/1
  ION multiply33/1(Kx) -> abc/dq-grid voltage4/1(iga)
  ION multiply36/1(Kx) -> abc/dq-grid voltage4/2(igb)
  ION multiply17/1(Kx) -> Inverse Park Transformation1/2
  softwave and hardwave protect/1(SFB) -> Subsystem1/5(SFB)
  Sum5/1 -> ION multiply44/1(x)
  Sum17/1 -> ION multiply45/1(x)
  Constant21/1 -> Sum5/2
  [Vpa] -> Sum5/1
  [ipa] -> ION multiply46/1(x)
  ION multiply46/1(Kx) -> Sum17/1
  Constant16/1 -> Sum17/2
  ION multiply44/1(Kx) -> Subsystem1/6(In1)
  ION multiply45/1(Kx) -> Subsystem1/7(In2)
  Constant18/1 -> PI-4/6(OV)
  [Kdv] -> PI-4/5(D)
  [Kiv] -> PI-4/4(I)
  [Kpv] -> PI-4/3(P)

== system Final_V620140905h5b_fuben1/Function-Call Subsystem3 ==
  function : TriggerPort  TriggerType=function-call
  Constant10 : Constant  OutDataTypeStr=fixdt(1,32,16)
  Integration 0 to maximal3 : Subsystem  mask{a=4}
      mask prompts: a "the maximal y"
  Memory Copy1 : idelinklib_common/Memory Copy  Priority=9  copyFrom=Specified source code symbol  copyFromAddressSource=Specify via dialog  copyFromAddress=hex2dec('200004')  copyFromSrcCode=data1  dataTypeFrom=int16  dataDimensionFrom=8  useOffsetFrom=off  offsetFromSrc=Specify via dialog  offsetFrom=0  strideFrom=1  copyTo=Output port  copyToAddressSource=Specify via dialog  copyToAddress=temp  copyToSrcCode=wave3  dataTypeTo=int16  useOffsetTo=off  offsetToSrc=Input port  offsetTo=0  strideTo=1  sampleTime=inf  useInitValue=off  initValueSrc=Specify constant value  initValue=bin2dec('00000000')  initValueSrcCode=myInitValueVariable  useAsMask=off  maskOperator=bitwise AND  useTermValue=off  termValue=bin2dec('00000000')  isRealtimeEnabled=off  emitCCBeforeWrite=off  CCBeforeWrite=/* Custom Code Before Write*/  emitCCAfterWrite=off  CCAfterWrite=/* Custom Code After Write*/  useDMACopy=off  enableBlockingMode=off
  Memory Copy2 : idelinklib_common/Memory Copy  Priority=9  copyFrom=Specified source code symbol  copyFromAddressSource=Specify via dialog  copyFromAddress=hex2dec('200004')  copyFromSrcCode=data2  dataTypeFrom=int16  dataDimensionFrom=8  useOffsetFrom=off  offsetFromSrc=Specify via dialog  offsetFrom=0  strideFrom=1  copyTo=Output port  copyToAddressSource=Specify via dialog  copyToAddress=temp  copyToSrcCode=wave3  dataTypeTo=int16  useOffsetTo=off  offsetToSrc=Input port  offsetTo=0  strideTo=1  sampleTime=inf  useInitValue=off  initValueSrc=Specify constant value  initValue=bin2dec('00000000')  initValueSrcCode=myInitValueVariable  useAsMask=off  maskOperator=bitwise AND  useTermValue=off  termValue=bin2dec('00000000')  isRealtimeEnabled=off  emitCCBeforeWrite=off  CCBeforeWrite=/* Custom Code Before Write*/  emitCCAfterWrite=off  CCAfterWrite=/* Custom Code After Write*/  useDMACopy=off  enableBlockingMode=off
  Memory Copy3 : idelinklib_common/Memory Copy  Priority=9  copyFrom=Specified source code symbol  copyFromAddressSource=Specify via dialog  copyFromAddress=hex2dec('200004')  copyFromSrcCode=data3  dataTypeFrom=int16  dataDimensionFrom=8  useOffsetFrom=off  offsetFromSrc=Specify via dialog  offsetFrom=0  strideFrom=1  copyTo=Output port  copyToAddressSource=Specify via dialog  copyToAddress=temp  copyToSrcCode=wave3  dataTypeTo=int16  useOffsetTo=off  offsetToSrc=Input port  offsetTo=0  strideTo=1  sampleTime=inf  useInitValue=off  initValueSrc=Specify constant value  initValue=bin2dec('00000000')  initValueSrcCode=myInitValueVariable  useAsMask=off  maskOperator=bitwise AND  useTermValue=off  termValue=bin2dec('00000000')  isRealtimeEnabled=off  emitCCBeforeWrite=off  CCBeforeWrite=/* Custom Code Before Write*/  emitCCAfterWrite=off  CCAfterWrite=/* Custom Code After Write*/  useDMACopy=off  enableBlockingMode=off
  Memory Copy7 : idelinklib_common/Memory Copy  Priority=9  copyFrom=Specified source code symbol  copyFromAddressSource=Specify via dialog  copyFromAddress=hex2dec('200004')  copyFromSrcCode=data  dataTypeFrom=int16  dataDimensionFrom=8  useOffsetFrom=off  offsetFromSrc=Specify via dialog  offsetFrom=0  strideFrom=1  copyTo=Output port  copyToAddressSource=Specify via dialog  copyToAddress=temp  copyToSrcCode=wave3  dataTypeTo=int16  useOffsetTo=off  offsetToSrc=Input port  offsetTo=0  strideTo=1  sampleTime=inf  useInitValue=off  initValueSrc=Specify constant value  initValue=bin2dec('00000000')  initValueSrcCode=myInitValueVariable  useAsMask=off  maskOperator=bitwise AND  useTermValue=off  termValue=bin2dec('00000000')  isRealtimeEnabled=off  emitCCBeforeWrite=off  CCBeforeWrite=/* Custom Code Before Write*/  emitCCAfterWrite=off  CCAfterWrite=/* Custom Code After Write*/  useDMACopy=off  enableBlockingMode=off
  Multiport Switch : MultiPortSwitch  Inputs=4  zeroidx=off
  SCI Transmit : c280xlib/SCI Transmit  sciModule=B  dataHead=''  dataTail=''  postInterrupt=off  numFifo=0
  wires:
  Constant10/1 -> Integration 0 to maximal3/1(x)
  Multiport Switch/1 -> SCI Transmit/1
  Memory Copy7/1 -> Multiport Switch/2
  Integration 0 to maximal3/1(y) -> Multiport Switch/1
  Memory Copy1/1 -> Multiport Switch/3
  Memory Copy2/1 -> Multiport Switch/4
  Memory Copy3/1 -> Multiport Switch/5

== system Final_V620140905h5b_fuben1/ION multiply1 ==
  x : Inport
  Constant2 : Constant  Value=x  OutDataTypeStr=fixdt(1,32,16)
  IQN x IQN : tiiqmathlib/IQN x IQN  multiplyOption=Multiply
  Kx : Outport
  wires:
  IQN x IQN/1 -> Kx/1
  x/1 -> IQN x IQN/1
  Constant2/1 -> IQN x IQN/2

== system Final_V620140905h5b_fuben1/ION multiply10 ==
  x : Inport
  Constant2 : Constant  Value=x  OutDataTypeStr=fixdt(1,32,16)
  IQN x IQN : tiiqmathlib/IQN x IQN  multiplyOption=Multiply
  Kx : Outport
  wires:
  IQN x IQN/1 -> Kx/1
  x/1 -> IQN x IQN/1
  Constant2/1 -> IQN x IQN/2

== system Final_V620140905h5b_fuben1/ION multiply11 ==
  x : Inport
  Constant2 : Constant  Value=x  OutDataTypeStr=fixdt(1,32,16)
  IQN x IQN : tiiqmathlib/IQN x IQN  multiplyOption=Multiply
  Kx : Outport
  wires:
  Constant2/1 -> IQN x IQN/2
  x/1 -> IQN x IQN/1
  IQN x IQN/1 -> Kx/1

== system Final_V620140905h5b_fuben1/ION multiply12 ==
  x : Inport
  Constant2 : Constant  Value=x  OutDataTypeStr=fixdt(1,32,16)
  IQN x IQN : tiiqmathlib/IQN x IQN  multiplyOption=Multiply
  Kx : Outport
  wires:
  IQN x IQN/1 -> Kx/1
  x/1 -> IQN x IQN/1
  Constant2/1 -> IQN x IQN/2

== system Final_V620140905h5b_fuben1/ION multiply13 ==
  x : Inport
  Constant2 : Constant  Value=x  OutDataTypeStr=fixdt(1,32,16)
  IQN x IQN : tiiqmathlib/IQN x IQN  multiplyOption=Multiply
  Kx : Outport
  wires:
  Constant2/1 -> IQN x IQN/2
  x/1 -> IQN x IQN/1
  IQN x IQN/1 -> Kx/1

== system Final_V620140905h5b_fuben1/ION multiply14 ==
  x : Inport
  Constant2 : Constant  Value=x  OutDataTypeStr=fixdt(1,32,16)
  IQN x IQN : tiiqmathlib/IQN x IQN  multiplyOption=Multiply
  Kx : Outport
  wires:
  IQN x IQN/1 -> Kx/1
  x/1 -> IQN x IQN/1
  Constant2/1 -> IQN x IQN/2

== system Final_V620140905h5b_fuben1/ION multiply15 ==
  x : Inport
  Constant2 : Constant  Value=x  OutDataTypeStr=fixdt(1,32,16)
  IQN x IQN : tiiqmathlib/IQN x IQN  multiplyOption=Multiply
  Kx : Outport
  wires:
  Constant2/1 -> IQN x IQN/2
  x/1 -> IQN x IQN/1
  IQN x IQN/1 -> Kx/1

== system Final_V620140905h5b_fuben1/ION multiply17 ==
  x : Inport
  Constant2 : Constant  Value=x  OutDataTypeStr=fixdt(1,32,16)
  IQN x IQN : tiiqmathlib/IQN x IQN  multiplyOption=Multiply
  Kx : Outport
  wires:
  Constant2/1 -> IQN x IQN/2
  x/1 -> IQN x IQN/1
  IQN x IQN/1 -> Kx/1

== system Final_V620140905h5b_fuben1/ION multiply18 ==
  x : Inport
  Constant2 : Constant  Value=x  OutDataTypeStr=fixdt(1,32,16)
  IQN x IQN : tiiqmathlib/IQN x IQN  multiplyOption=Multiply
  Kx : Outport
  wires:
  IQN x IQN/1 -> Kx/1
  x/1 -> IQN x IQN/1
  Constant2/1 -> IQN x IQN/2

== system Final_V620140905h5b_fuben1/ION multiply19 ==
  x : Inport
  Constant2 : Constant  Value=x  OutDataTypeStr=fixdt(1,32,16)
  IQN x IQN : tiiqmathlib/IQN x IQN  multiplyOption=Multiply
  Kx : Outport
  wires:
  Constant2/1 -> IQN x IQN/2
  x/1 -> IQN x IQN/1
  IQN x IQN/1 -> Kx/1

== system Final_V620140905h5b_fuben1/ION multiply2 ==
  x : Inport
  Constant2 : Constant  Value=x  OutDataTypeStr=fixdt(1,32,16)
  IQN x IQN : tiiqmathlib/IQN x IQN  multiplyOption=Multiply
  Kx : Outport
  wires:
  Constant2/1 -> IQN x IQN/2
  x/1 -> IQN x IQN/1
  IQN x IQN/1 -> Kx/1

== system Final_V620140905h5b_fuben1/ION multiply20 ==
  x : Inport
  Constant2 : Constant  Value=x  OutDataTypeStr=fixdt(1,32,16)
  IQN x IQN : tiiqmathlib/IQN x IQN  multiplyOption=Multiply
  Kx : Outport
  wires:
  IQN x IQN/1 -> Kx/1
  x/1 -> IQN x IQN/1
  Constant2/1 -> IQN x IQN/2

== system Final_V620140905h5b_fuben1/ION multiply21 ==
  x : Inport
  Constant2 : Constant  Value=x  OutDataTypeStr=fixdt(1,32,16)
  IQN x IQN : tiiqmathlib/IQN x IQN  multiplyOption=Multiply
  Kx : Outport
  wires:
  Constant2/1 -> IQN x IQN/2
  x/1 -> IQN x IQN/1
  IQN x IQN/1 -> Kx/1

== system Final_V620140905h5b_fuben1/ION multiply22 ==
  x : Inport
  Constant2 : Constant  Value=x  OutDataTypeStr=fixdt(1,32,16)
  IQN x IQN : tiiqmathlib/IQN x IQN  multiplyOption=Multiply
  Kx : Outport
  wires:
  IQN x IQN/1 -> Kx/1
  x/1 -> IQN x IQN/1
  Constant2/1 -> IQN x IQN/2

== system Final_V620140905h5b_fuben1/ION multiply23 ==
  x : Inport
  Constant2 : Constant  Value=x  OutDataTypeStr=fixdt(1,32,16)
  IQN x IQN : tiiqmathlib/IQN x IQN  multiplyOption=Multiply
  Kx : Outport
  wires:
  Constant2/1 -> IQN x IQN/2
  x/1 -> IQN x IQN/1
  IQN x IQN/1 -> Kx/1

== system Final_V620140905h5b_fuben1/ION multiply24 ==
  x : Inport
  Constant2 : Constant  Value=x  OutDataTypeStr=fixdt(1,32,16)
  IQN x IQN : tiiqmathlib/IQN x IQN  multiplyOption=Multiply
  Kx : Outport
  wires:
  IQN x IQN/1 -> Kx/1
  x/1 -> IQN x IQN/1
  Constant2/1 -> IQN x IQN/2

== system Final_V620140905h5b_fuben1/ION multiply26 ==
  x : Inport
  Constant2 : Constant  Value=x  OutDataTypeStr=fixdt(1,32,16)
  IQN x IQN : tiiqmathlib/IQN x IQN  multiplyOption=Multiply
  Kx : Outport
  wires:
  IQN x IQN/1 -> Kx/1
  x/1 -> IQN x IQN/1
  Constant2/1 -> IQN x IQN/2

== system Final_V620140905h5b_fuben1/ION multiply27 ==
  x : Inport
  Constant2 : Constant  Value=x  OutDataTypeStr=fixdt(1,32,16)
  IQN x IQN : tiiqmathlib/IQN x IQN  multiplyOption=Multiply
  Kx : Outport
  wires:
  Constant2/1 -> IQN x IQN/2
  x/1 -> IQN x IQN/1
  IQN x IQN/1 -> Kx/1

== system Final_V620140905h5b_fuben1/ION multiply28 ==
  x : Inport
  Constant2 : Constant  Value=x  OutDataTypeStr=fixdt(1,32,16)
  IQN x IQN : tiiqmathlib/IQN x IQN  multiplyOption=Multiply
  Kx : Outport
  wires:
  IQN x IQN/1 -> Kx/1
  x/1 -> IQN x IQN/1
  Constant2/1 -> IQN x IQN/2

== system Final_V620140905h5b_fuben1/ION multiply29 ==
  x : Inport
  Constant2 : Constant  Value=x  OutDataTypeStr=fixdt(1,32,16)
  IQN x IQN : tiiqmathlib/IQN x IQN  multiplyOption=Multiply
  Kx : Outport
  wires:
  Constant2/1 -> IQN x IQN/2
  x/1 -> IQN x IQN/1
  IQN x IQN/1 -> Kx/1

== system Final_V620140905h5b_fuben1/ION multiply3 ==
  x : Inport
  Constant2 : Constant  Value=x  OutDataTypeStr=fixdt(1,32,16)
  IQN x IQN : tiiqmathlib/IQN x IQN  multiplyOption=Multiply
  Kx : Outport
  wires:
  IQN x IQN/1 -> Kx/1
  x/1 -> IQN x IQN/1
  Constant2/1 -> IQN x IQN/2

== system Final_V620140905h5b_fuben1/ION multiply30 ==
  x : Inport
  Constant2 : Constant  Value=x  OutDataTypeStr=fixdt(1,32,16)
  IQN x IQN : tiiqmathlib/IQN x IQN  multiplyOption=Multiply
  Kx : Outport
  wires:
  IQN x IQN/1 -> Kx/1
  x/1 -> IQN x IQN/1
  Constant2/1 -> IQN x IQN/2

== system Final_V620140905h5b_fuben1/ION multiply31 ==
  x : Inport
  Constant2 : Constant  Value=x  OutDataTypeStr=fixdt(1,32,16)
  IQN x IQN : tiiqmathlib/IQN x IQN  multiplyOption=Multiply
  Kx : Outport
  wires:
  Constant2/1 -> IQN x IQN/2
  x/1 -> IQN x IQN/1
  IQN x IQN/1 -> Kx/1

== system Final_V620140905h5b_fuben1/ION multiply32 ==
  x : Inport
  Constant2 : Constant  Value=x  OutDataTypeStr=fixdt(1,32,16)
  IQN x IQN : tiiqmathlib/IQN x IQN  multiplyOption=Multiply
  Kx : Outport
  wires:
  IQN x IQN/1 -> Kx/1
  x/1 -> IQN x IQN/1
  Constant2/1 -> IQN x IQN/2

== system Final_V620140905h5b_fuben1/ION multiply33 ==
  x : Inport
  Constant2 : Constant  Value=x  OutDataTypeStr=fixdt(1,32,16)
  IQN x IQN : tiiqmathlib/IQN x IQN  multiplyOption=Multiply
  Kx : Outport
  wires:
  Constant2/1 -> IQN x IQN/2
  x/1 -> IQN x IQN/1
  IQN x IQN/1 -> Kx/1

== system Final_V620140905h5b_fuben1/ION multiply34 ==
  x : Inport
  Constant2 : Constant  Value=x  OutDataTypeStr=fixdt(1,32,16)
  IQN x IQN : tiiqmathlib/IQN x IQN  multiplyOption=Multiply
  Kx : Outport
  wires:
  IQN x IQN/1 -> Kx/1
  x/1 -> IQN x IQN/1
  Constant2/1 -> IQN x IQN/2

== system Final_V620140905h5b_fuben1/ION multiply8 ==
  x : Inport
  Constant2 : Constant  Value=x  OutDataTypeStr=fixdt(1,32,16)
  IQN x IQN : tiiqmathlib/IQN x IQN  multiplyOption=Multiply
  Kx : Outport
  wires:
  IQN x IQN/1 -> Kx/1
  x/1 -> IQN x IQN/1
  Constant2/1 -> IQN x IQN/2

== system Final_V620140905h5b_fuben1/ION multiply9 ==
  x : Inport
  Constant2 : Constant  Value=x  OutDataTypeStr=fixdt(1,32,16)
  IQN x IQN : tiiqmathlib/IQN x IQN  multiplyOption=Multiply
  Kx : Outport
  wires:
  Constant2/1 -> IQN x IQN/2
  x/1 -> IQN x IQN/1
  IQN x IQN/1 -> Kx/1
